simulink model "chap1_7"  (Simulink 3.00)
settings: Solver=ode4  StartTime=0.0  StopTime=1.0  RelTol=1e-3
undefined symbols (not defined in the file or in its folder): chap1_7f
settings Model: SaveTime=off  SaveOutput=off  Decimation=100

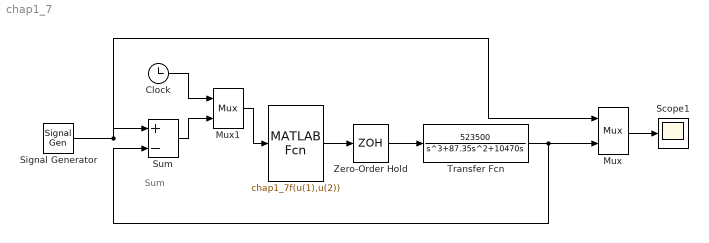
== system chap1_7 ==
  note: Sum
  "    " : MATLABFcn  MATLABFcn=chap1_7f(u(1),u(2))  OutputWidth=-1  OutputSignalType=auto
  Clock : Clock
      settings: DisplayTime=off  Decimation=10
  Mux : Mux  Inputs=2
      settings: DisplayOption=none
  Mux1 : Mux  Inputs=2
      settings: DisplayOption=none
  Scope1 : Scope
      settings: TimeRange=0.2  YMin=-0.051  YMax=-0.041  SaveToWorkspace=off  SaveName=ScopeData  MaxRows=50000  Decimation=0.001  SampleInput=on  SampleTime=0.001
  Signal Generator : SignalGenerator  WaveForm=sine  Amplitude=0.05  Frequency=1  Units=Hertz
  Sum : Sum  Inputs=|+-  SaturateOnIntegerOverflow=on
  Transfer Fcn : TransferFcn  Numerator=[523500]  Denominator=[1 87.35 10470 0]
  Zero-Order Hold : ZeroOrderHold  SampleTime=0.001
  wires:
  Mux/1 -> Scope1/1
  Transfer Fcn/1 -> Sum/2, Mux/2
  Signal Generator/1 -> Sum/1, Mux/1
  Clock/1 -> Mux1/1
  Sum/1 -> Mux1/2
  Mux1/1 -> "    "/1
  Zero-Order Hold/1 -> Transfer Fcn/1
  "    "/1 -> Zero-Order Hold/1
